simulink model "TP3"  (R2022b)
settings: Solver=VariableStepAuto  StartTime=0.0  StopTime=10.0  RelTol=1e-3
InitFcn:
  | U0 = 220;
  | phy = pi/4;
  | 
  | R = 0.895;
  | L0 = 12.16e-3;
  | J = 0.2;
  | K = 0.9;
  | p = 3;
  | phi_f = K/p;
StartFcn:
  | TP3_config
values from neighbouring files (symbols this model uses):
  Cr = 0    [TP3_config.m]
settings Model: Creator=Youssef ABLALI  LastModifiedBy=Youssef ABLALI

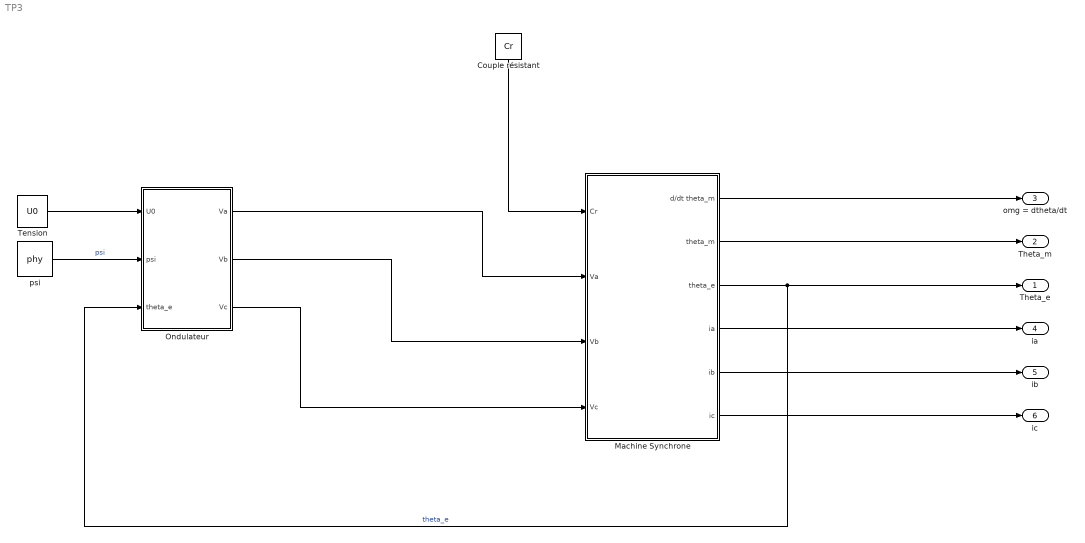
== system TP3 ==
  Couple résistant : Constant  Value=Cr
  Machine Synchrone : Subsystem
  "Ondulateur " : Subsystem
  Tension : Constant  Value=U0
  psi : Constant  Value=phy
  Theta_e : Outport
  Theta_m : Outport  Port=2
  omg = dtheta/dt : Outport  Port=3
  ia : Outport  Port=4
  ib : Outport  Port=5
  ic : Outport  Port=6
  wires:
  Couple résistant/1 -> Machine Synchrone/1(Cr)
  Machine Synchrone/1(d/dt theta_m) -> omg = dtheta/dt/1
  Machine Synchrone/2(theta_m) -> Theta_m/1
  Machine Synchrone/4(ia) -> ia/1
  Machine Synchrone/5(ib) -> ib/1
  Machine Synchrone/6(ic) -> ic/1
  Machine Synchrone/3(theta_e) -> "Ondulateur "/3(theta_e), Theta_e/1  "theta_e"
  Tension/1 -> "Ondulateur "/1(U0)
  psi/1 -> "Ondulateur "/2(psi)  "psi"
  "Ondulateur "/1(Va) -> Machine Synchrone/2(Va)
  "Ondulateur "/2(Vb) -> Machine Synchrone/3(Vb)
  "Ondulateur "/3(Vc) -> Machine Synchrone/4(Vc)

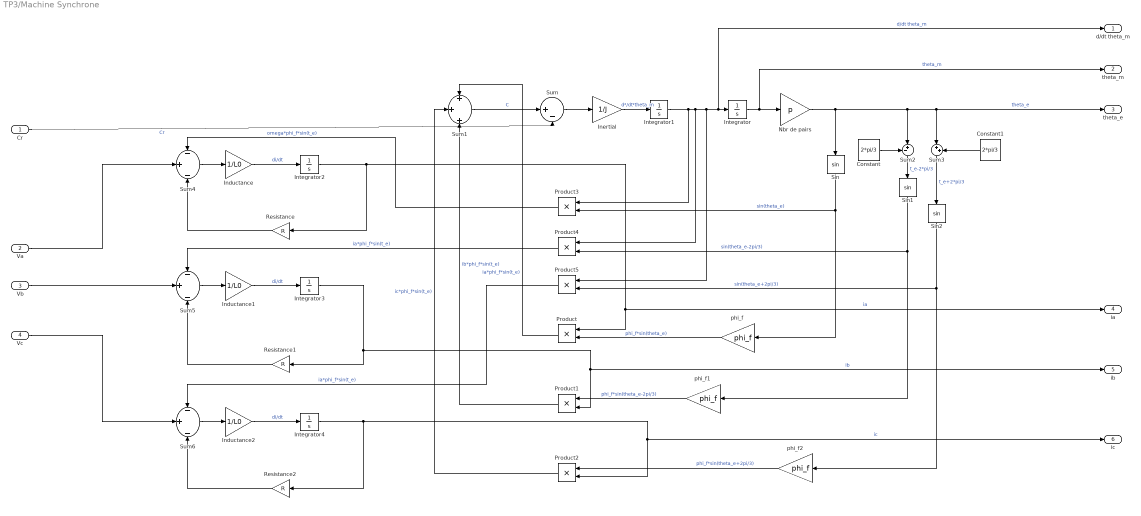
== system TP3/Machine Synchrone ==
  Cr : Inport
  Va : Inport  Port=2
  Vb : Inport  Port=3
  Vc : Inport  Port=4
  Constant : Constant  Value=2*pi/3
  Constant1 : Constant  Value=2*pi/3
  Inductance : Gain  Gain=1/L0
  Inductance1 : Gain  Gain=1/L0
  Inductance2 : Gain  Gain=1/L0
  Inertial : Gain  Gain=1/J
  Integrator{,1..4} (5 alike) : Integrator
  Nbr de pairs : Gain  Gain=p
  Product{,1..5} (6 alike) : Product
  Resistance : Gain  Gain=R
  Resistance1 : Gain  Gain=R
  Resistance2 : Gain  Gain=R
  Sin : Trigonometry
  Sin1 : Trigonometry
  Sin2 : Trigonometry
  Sum : Sum  Inputs=|+-
  Sum1 : Sum  Inputs=+|+|+
  Sum2 : Sum  Inputs=-+|
  Sum3 : Sum  Inputs=|++
  Sum4 : Sum  Inputs=-|+|-
  Sum5 : Sum  Inputs=-|+|-
  Sum6 : Sum  Inputs=-|+|-
  phi_f : Gain  Gain=phi_f
  phi_f1 : Gain  Gain=phi_f
  phi_f2 : Gain  Gain=phi_f
  d/dt theta_m : Outport
  theta_m : Outport  Port=2
  theta_e : Outport  Port=3
  ia : Outport  Port=4
  ib : Outport  Port=5
  ic : Outport  Port=6
  wires:
  Integrator2/1 -> ia/1, Product/1, Resistance/1  "ia"
  Integrator/1 -> theta_m/1, Nbr de pairs/1  "theta_m"
  Resistance2/1 -> Sum6/3
  Integrator1/1 -> Product3/1, Product4/1, Product5/1, d/dt theta_m/1, Integrator/1  "d/dt theta_m"
  Resistance1/1 -> Sum5/3
  Sum/1 -> Inertial/1
  Sin2/1 -> Product5/2, phi_f2/1  "sin(theta_e+2pi/3)"
  Integrator4/1 -> Resistance2/1, ic/1, Product2/2  "ic"
  Sum1/1 -> Sum/1  "C"
  Sin/1 -> Product3/2, phi_f/1  "sin(theta_e)"
  Product/1 -> Sum1/1  "ia*phi_f*sin(t_e)"
  Sum4/1 -> Inductance/1
  phi_f2/1 -> Product2/1  "phi_f*sin(theta_e+2pi/3)"
  Inductance/1 -> Integrator2/1  "di/dt"
  Nbr de pairs/1 -> Sum2/2, theta_e/1, Sum3/1, Sin/1  "theta_e"
  Sum3/1 -> Sin2/1  "t_e+2*pi/3"
  Resistance/1 -> Sum4/3
  Inductance1/1 -> Integrator3/1  "di/dt"
  phi_f1/1 -> Product1/1  "phi_f*sin(theta_e-2pi/3)"
  Sin1/1 -> Product4/2, phi_f1/1  "sin(theta_e-2pi/3)"
  Sum5/1 -> Inductance1/1
  phi_f/1 -> Product/2  "phi_f*sin(theta_e)"
  Constant/1 -> Sum2/1
  Integrator3/1 -> Resistance1/1, ib/1, Product1/2  "ib"
  Sum2/1 -> Sin1/1  "t_e-2*pi/3"
  Product5/1 -> Sum6/1  "ia*phi_f*sin(t_e)"
  Vb/1 -> Sum5/2
  Va/1 -> Sum4/2
  Product2/1 -> Sum1/2  "ic*phi_f*sin(t_e)"
  Product1/1 -> Sum1/3  "ib*phi_f*sin(t_e)"
  Cr/1 -> Sum/2  "Cr"
  Constant1/1 -> Sum3/2
  Sum6/1 -> Inductance2/1
  Product4/1 -> Sum5/1  "ia*phi_f*sin(t_e)"
  Inductance2/1 -> Integrator4/1  "di/dt"
  Product3/1 -> Sum4/1  "omega*phi_f*sin(t_e)"
  Vc/1 -> Sum6/2
  Inertial/1 -> Integrator1/1  "d²/dt²theta_m"

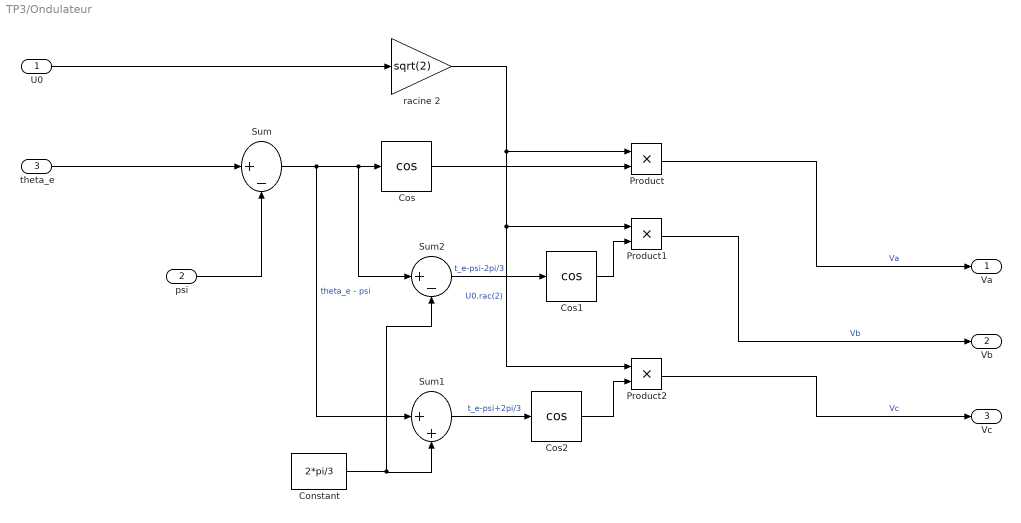
== system TP3/Ondulateur  ==
  U0 : Inport
  psi : Inport  Port=2
  theta_e : Inport  Port=3
  Constant : Constant  Value=2*pi/3
  Cos : Trigonometry  Operator=cos
  Cos1 : Trigonometry  Operator=cos
  Cos2 : Trigonometry  Operator=cos
  Product : Product
  Product1 : Product
  Product2 : Product
  Sum : Sum  Inputs=|+-
  Sum1 : Sum  Inputs=|++
  Sum2 : Sum  Inputs=|+-
  racine 2 : Gain  Gain=sqrt(2)
  Va : Outport
  Vb : Outport  Port=2
  Vc : Outport  Port=3
  wires:
  Constant/1 -> Sum2/2, Sum1/2
  Sum/1 -> Sum1/1, Sum2/1, Cos/1  "theta_e - psi"
  Cos1/1 -> Product1/2
  Cos/1 -> Product/2
  racine 2/1 -> Product2/1, Product1/1, Product/1  "U0.rac(2)"
  Sum1/1 -> Cos2/1  "t_e-psi+2pi/3"
  Cos2/1 -> Product2/2
  Sum2/1 -> Cos1/1  "t_e-psi-2pi/3"
  Product/1 -> Va/1  "Va"
  psi/1 -> Sum/2
  U0/1 -> racine 2/1
  Product2/1 -> Vc/1  "Vc"
  Product1/1 -> Vb/1  "Vb"
  theta_e/1 -> Sum/1
